simulink library "cmd_command_shaper_lib"  (R2016b)
settings: Solver=ode45  StartTime=0.0  StopTime=10.0  RelTol=1e-3  EnableMultiTasking=on
libraries: math_utils x4
settings Model: Creator=rhnakamu  LastModifiedBy=jfusco1
settings DataIOCC: LimitDataPoints=on  SaveFormat=Array
settings OptimizationCC: LifeSpan=inf
settings DebuggingCC: AllowSymbolicDim=off  SFUnexpectedBacktrackingDiag=warning  SFNoUnconditionalDefaultTransitionDiag=warning  SFExecutionAtInitializationDiag=none
settings HardwareCC: ProdBitPerPointer=32  ProdBitPerSizeT=32  ProdBitPerPtrDiffT=32  ProdLargestAtomicFloat=None  ProdIntDivRoundTo=Undefined  ProdEndianess=Unspecified  ProdWordSize=32  ProdHWDeviceType=32-bit Generic
settings ModelReferenceCC: PropagateSignalLabelsOutOfModel=off
settings GRTTargetCC: TargetLangStandard=C89/C90 (ANSI)  GeneratePreprocessorConditionals=Disable all
settings ConfigComp: CovMetricSettings=dw  CovHtmlReporting=on  CovSaveCumulativeToWorkspaceVar=on  CovSaveSingleToWorkspaceVar=on  CovExternalEMLEnable=off

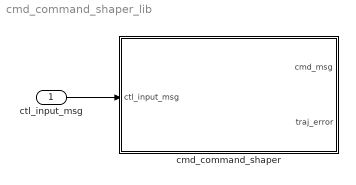
== system cmd_command_shaper_lib ==
  ctl_input_msg : Inport  OutDataTypeStr=Bus: ctl_input_msg
  cmd_command_shaper : Subsystem
  wires:
  ctl_input_msg/1 -> cmd_command_shaper/1(ctl_input_msg)

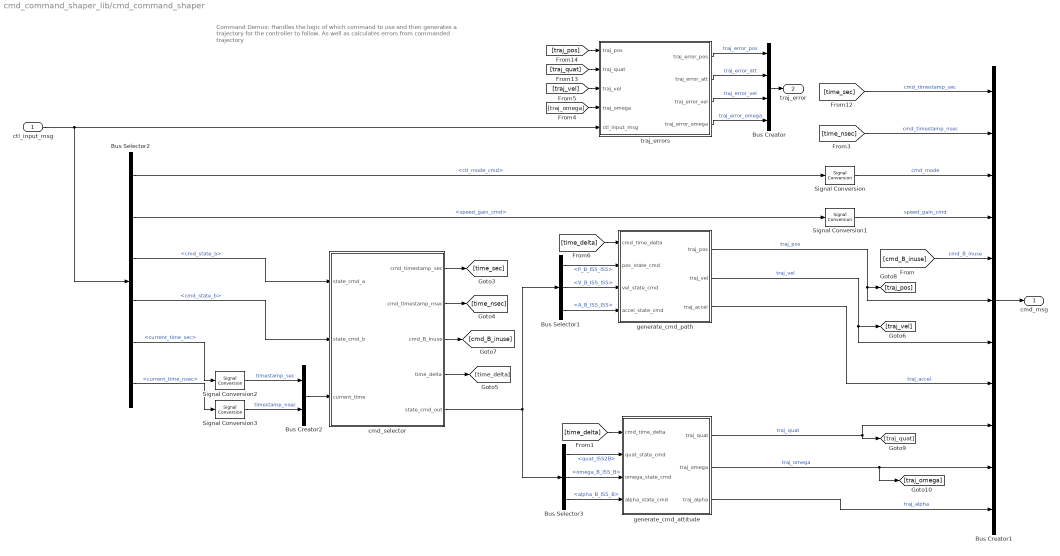
== system cmd_command_shaper_lib/cmd_command_shaper ==
  note: Command Demux:
      | Handles the logic of which command to use and then generates a trajectory for the controller to follow.
      | As well as calculates errors from commanded trajectory
  ctl_input_msg : Inport  OutDataTypeStr=Bus: ctl_input_msg
  Bus Creator : BusCreator  Inputs=4
  Bus Creator1 : BusCreator  Inputs=11  OutDataTypeStr=Bus: cmd_msg  NonVirtualBus=on
  Bus Creator2 : BusCreator  Inputs=2  OutDataTypeStr=Bus: ex_time_msg  NonVirtualBus=on
  Bus Selector1 : BusSelector  OutputSignals=P_B_ISS_ISS,V_B_ISS_ISS,A_B_ISS_ISS
  Bus Selector2 : BusSelector  OutputSignals=ctl_mode_cmd,speed_gain_cmd,cmd_state_a,cmd_state_b,current_time_sec,current_time_nsec
  Bus Selector3 : BusSelector  OutputSignals=quat_ISS2B,omega_B_ISS_B,alpha_B_ISS_B
  Signal Conversion{,1..3} (4 alike) : SignalConversion  OverrideOpt=off
  cmd_selector : Subsystem
  generate_cmd_attitude : Subsystem
  generate_cmd_path : Subsystem
  traj_errors : Subsystem
  cmd_msg : Outport  OutDataTypeStr=Bus: cmd_msg
  traj_error : Outport  Port=2
  wires:
  generate_cmd_attitude/1(traj_quat) -> Bus Creator1/9, [traj_quat]  "traj_quat"
  generate_cmd_attitude/2(traj_omega) -> [traj_omega], Bus Creator1/10  "traj_omega"
  generate_cmd_attitude/3(traj_alpha) -> Bus Creator1/11  "traj_alpha"
  generate_cmd_path/2(traj_vel) -> Bus Creator1/7, [traj_vel]  "traj_vel"
  generate_cmd_path/3(traj_accel) -> Bus Creator1/8  "traj_accel"
  generate_cmd_path/1(traj_pos) -> Bus Creator1/6, [traj_pos]  "traj_pos"
  [cmd_B_inuse] -> Bus Creator1/5  "cmd_B_inuse"
  cmd_selector/3(cmd_B_inuse) -> [cmd_B_inuse]
  [traj_pos] -> traj_errors/1(traj_pos)
  [traj_quat] -> traj_errors/2(traj_quat)
  Signal Conversion/1 -> Bus Creator1/3  "cmd_mode"
  Bus Selector2/1 -> Signal Conversion/1  "<ctl_mode_cmd>"
  [time_nsec] -> Bus Creator1/2  "cmd_timestamp_nsec"
  [time_sec] -> Bus Creator1/1  "cmd_timestamp_sec"
  Bus Creator1/1 -> cmd_msg/1
  Bus Creator2/1 -> cmd_selector/3(current_time)
  cmd_selector/4(time_delta) -> [time_delta]
  [time_delta] -> generate_cmd_path/1(cmd_time_delta)
  cmd_selector/1(cmd_timestamp_sec) -> [time_sec]
  cmd_selector/2(cmd_timestamp_nsec) -> [time_nsec]
  ctl_input_msg/1 -> traj_errors/5(ctl_input_msg), Bus Selector2/1
  cmd_selector/5(state_cmd_out) -> Bus Selector1/1, Bus Selector3/1
  [traj_vel] -> traj_errors/3(traj_vel)
  [traj_omega] -> traj_errors/4(traj_omega)
  traj_errors/1(traj_error_pos) -> Bus Creator/1  "traj_error_pos"
  traj_errors/2(traj_error_att) -> Bus Creator/2  "traj_error_att"
  traj_errors/3(traj_error_vel) -> Bus Creator/3  "traj_error_vel"
  traj_errors/4(traj_error_omega) -> Bus Creator/4  "traj_error_omega"
  Bus Creator/1 -> traj_error/1
  Bus Selector1/2 -> generate_cmd_path/3(vel_state_cmd)  "<V_B_ISS_ISS>"
  Bus Selector1/1 -> generate_cmd_path/2(pos_state_cmd)  "<P_B_ISS_ISS>"
  Bus Selector1/3 -> generate_cmd_path/4(accel_state_cmd)  "<A_B_ISS_ISS>"
  [time_delta] -> generate_cmd_attitude/1(cmd_time_delta)
  Bus Selector3/2 -> generate_cmd_attitude/3(omega_state_cmd)  "<omega_B_ISS_B>"
  Bus Selector3/1 -> generate_cmd_attitude/2(quat_state_cmd)  "<quat_ISS2B>"
  Bus Selector3/3 -> generate_cmd_attitude/4(alpha_state_cmd)  "<alpha_B_ISS_B>"
  Bus Selector2/3 -> cmd_selector/1(state_cmd_a)  "<cmd_state_a>"
  Bus Selector2/4 -> cmd_selector/2(state_cmd_b)  "<cmd_state_b>"
  Signal Conversion1/1 -> Bus Creator1/4  "speed_gain_cmd"
  Bus Selector2/2 -> Signal Conversion1/1  "<speed_gain_cmd>"
  Signal Conversion2/1 -> Bus Creator2/1  "timestamp_sec"
  Signal Conversion3/1 -> Bus Creator2/2  "timestamp_nsec"
  Bus Selector2/5 -> Signal Conversion2/1  "<current_time_sec>"
  Bus Selector2/6 -> Signal Conversion3/1  "<current_time_nsec>"

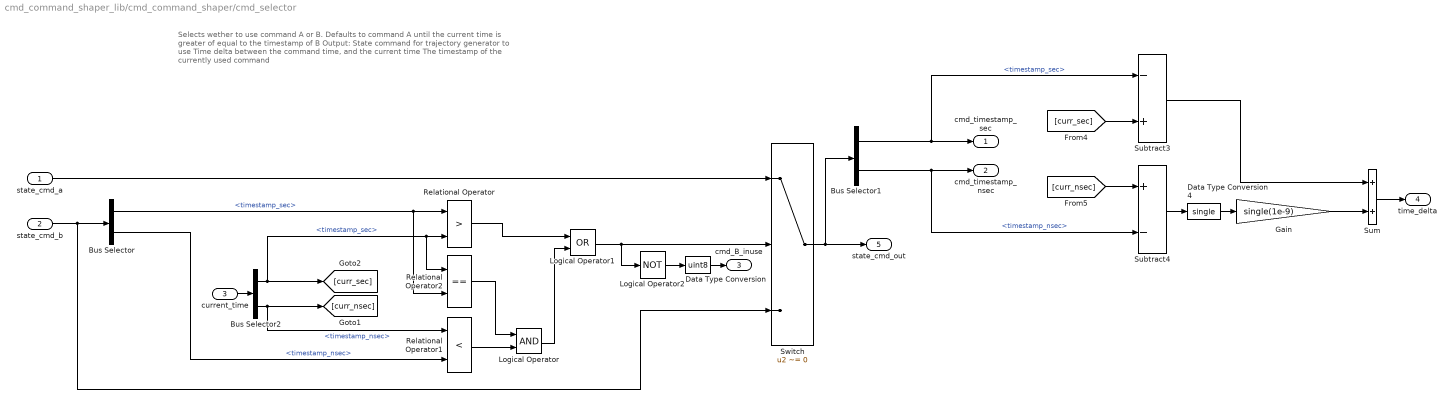
== system cmd_command_shaper_lib/cmd_command_shaper/cmd_selector ==
  note: Selects wether to use command A or B.
      | Defaults to command A until the current time is greater of equal to the timestamp of B
      |
      | Output:
      | 	State command for trajectory generator to use
      | 	Time delta between the command time, and the current time
      | 	The timestamp of the currently used command
  state_cmd_a : Inport
  state_cmd_b : Inport  Port=2
  current_time : Inport  Port=3
  Bus Selector : BusSelector  OutputSignals=timestamp_sec,timestamp_nsec
  Bus Selector1 : BusSelector  OutputSignals=timestamp_sec,timestamp_nsec
  Bus Selector2 : BusSelector  OutputSignals=timestamp_sec,timestamp_nsec
  Data Type Conversion : DataTypeConversion  OutDataTypeStr=uint8
  Data Type Conversion4 : DataTypeConversion  OutDataTypeStr=single
  Gain : Gain  Gain=single(1e-9)
  Logical Operator : Logic  AllPortsSameDT=off  OutDataTypeStr=boolean
  Logical Operator1 : Logic  Operator=OR  AllPortsSameDT=off  OutDataTypeStr=boolean
  Logical Operator2 : Logic  Operator=NOT  AllPortsSameDT=off  OutDataTypeStr=boolean
  Relational Operator : RelationalOperator  Operator=>  OutDataTypeStr=boolean  RndMeth=Nearest
  Relational Operator1 : RelationalOperator  Operator=<  OutDataTypeStr=boolean  RndMeth=Nearest
  Relational Operator2 : RelationalOperator  Operator===  OutDataTypeStr=boolean  RndMeth=Nearest
  Subtract3 : Sum  Inputs=-+  OutDataTypeStr=int32
      settings: AttributesFormatString=Out Type: %<OutDataTypeStr>
  Subtract4 : Sum  Inputs=+-  OutDataTypeStr=int32
      settings: AttributesFormatString=Out Type: %<OutDataTypeStr>
  Sum : Sum
  Switch : Switch  Criteria=u2 ~= 0
  cmd_timestamp_sec : Outport
  cmd_timestamp_nsec : Outport  Port=2
  cmd_B_inuse : Outport  Port=3
  time_delta : Outport  Port=4
  state_cmd_out : Outport  Port=5
  wires:
  Data Type Conversion/1 -> cmd_B_inuse/1
  Logical Operator2/1 -> Data Type Conversion/1
  Bus Selector1/2 -> cmd_timestamp_nsec/1, Subtract4/2  "<timestamp_nsec>"
  Bus Selector1/1 -> cmd_timestamp_sec/1, Subtract3/1  "<timestamp_sec>"
  Bus Selector/2 -> Relational Operator1/2  "<timestamp_nsec>"
  Bus Selector/1 -> Relational Operator/1, Relational Operator2/2  "<timestamp_sec>"
  Logical Operator1/1 -> Switch/2, Logical Operator2/1
  Subtract4/1 -> Data Type Conversion4/1
  [curr_sec] -> Subtract3/2
  [curr_nsec] -> Subtract4/1
  Sum/1 -> time_delta/1
  Data Type Conversion4/1 -> Gain/1
  Gain/1 -> Sum/2
  Subtract3/1 -> Sum/1
  Switch/1 -> Bus Selector1/1, state_cmd_out/1
  current_time/1 -> Bus Selector2/1
  Relational Operator/1 -> Logical Operator1/1
  Logical Operator/1 -> Logical Operator1/2
  Relational Operator2/1 -> Logical Operator/1
  Relational Operator1/1 -> Logical Operator/2
  Bus Selector2/1 -> [curr_sec], Relational Operator/2, Relational Operator2/1  "<timestamp_sec>"
  Bus Selector2/2 -> [curr_nsec], Relational Operator1/1  "<timestamp_nsec>"
  state_cmd_a/1 -> Switch/1
  state_cmd_b/1 -> Bus Selector/1, Switch/3

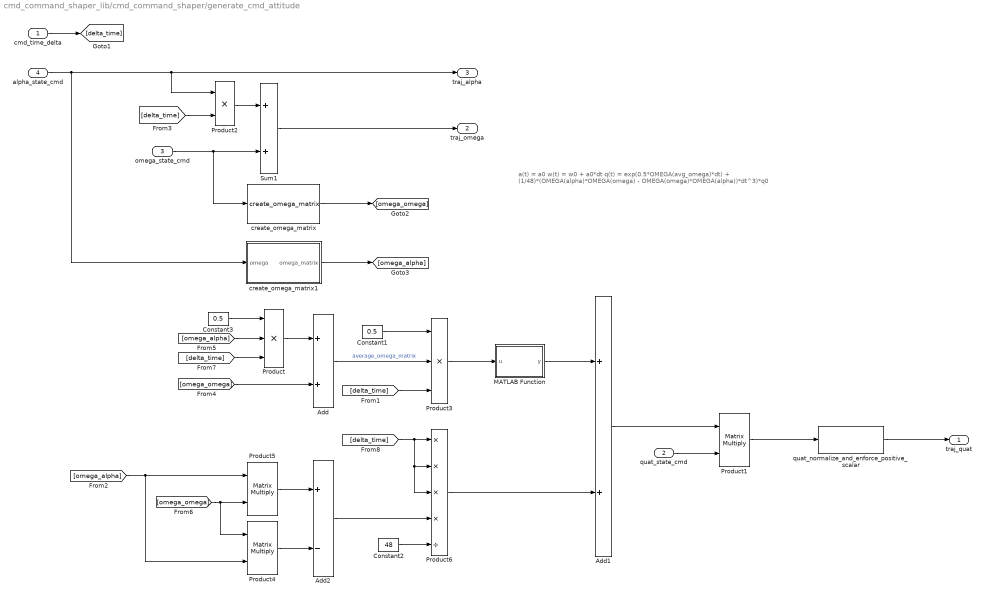
== system cmd_command_shaper_lib/cmd_command_shaper/generate_cmd_attitude ==
  note: a(t) = a0
      | w(t) = w0 + a0*dt
      | q(t) = exp(0.5*OMEGA(avg_omega)*dt) + (1/48)*(OMEGA(alpha)*OMEGA(omega) - OMEGA(omega)*OMEGA(alpha))*dt^3)*q0
  cmd_time_delta : Inport
  quat_state_cmd : Inport  Port=2
  omega_state_cmd : Inport  Port=3
  alpha_state_cmd : Inport  Port=4
  Add : Sum
  Add1 : Sum
  Add2 : Sum  Inputs=+-
  Constant1 : Constant  Value=0.5  OutDataTypeStr=Inherit: Inherit via back propagation
  Constant2 : Constant  Value=48  OutDataTypeStr=Inherit: Inherit via back propagation
  Constant3 : Constant  Value=0.5  OutDataTypeStr=Inherit: Inherit via back propagation
  MATLAB Function : MATLAB Function  TreatAsAtomicUnit=on
  Product : Product  Inputs=3
  Product1 : Product  Multiplication=Matrix(*)  RndMeth=Zero
  Product2 : Product  RndMeth=Zero  InputSameDT=on  OutDataTypeStr=Inherit: Same as first input
  Product3 : Product  Inputs=3
  Product4 : Product  Multiplication=Matrix(*)  RndMeth=Zero
  Product5 : Product  Multiplication=Matrix(*)  RndMeth=Zero
  Product6 : Product  Inputs=****/
  Sum1 : Sum
  create_omega_matrix : math_utils/create_omega_matrix  SystemSampleTime=-1
  create_omega_matrix1 : Subsystem
      mask Display: disp('\Omega(\omega)', 'tex', 'on');
  quat_normalize_and_enforce_positive_scalar : math_utils/quat_normalize_and_enforce_positive_scalar
  traj_quat : Outport
  traj_omega : Outport  Port=2
  traj_alpha : Outport  Port=3
  wires:
  Constant3/1 -> Product/1
  alpha_state_cmd/1 -> create_omega_matrix1/1(omega), Product2/1, traj_alpha/1
  Add1/1 -> Product1/1
  quat_state_cmd/1 -> Product1/2
  omega_state_cmd/1 -> create_omega_matrix/1, Sum1/2
  [delta_time] -> Product/3
  Product/1 -> Add/1
  Constant1/1 -> Product3/1
  Add/1 -> Product3/2  "average_omega_matrix"
  [delta_time] -> Product3/3
  Product3/1 -> MATLAB Function/1(u)
  MATLAB Function/1(y) -> Add1/1
  create_omega_matrix/1 -> [omega_omega]
  [omega_omega] -> Add/2
  [omega_alpha] -> Product/2
  create_omega_matrix1/1(omega_matrix) -> [omega_alpha]
  [omega_alpha] -> Product4/2, Product5/1
  Product5/1 -> Add2/1
  Product4/1 -> Add2/2
  [omega_omega] -> Product4/1, Product5/2
  Add2/1 -> Product6/4
  Constant2/1 -> Product6/5
  [delta_time] -> Product6/1, Product6/2, Product6/3
  Product6/1 -> Add1/2
  [delta_time] -> Product2/2
  cmd_time_delta/1 -> [delta_time]
  quat_normalize_and_enforce_positive_scalar/1 -> traj_quat/1
  Sum1/1 -> traj_omega/1
  Product2/1 -> Sum1/1
  Product1/1 -> quat_normalize_and_enforce_positive_scalar/1

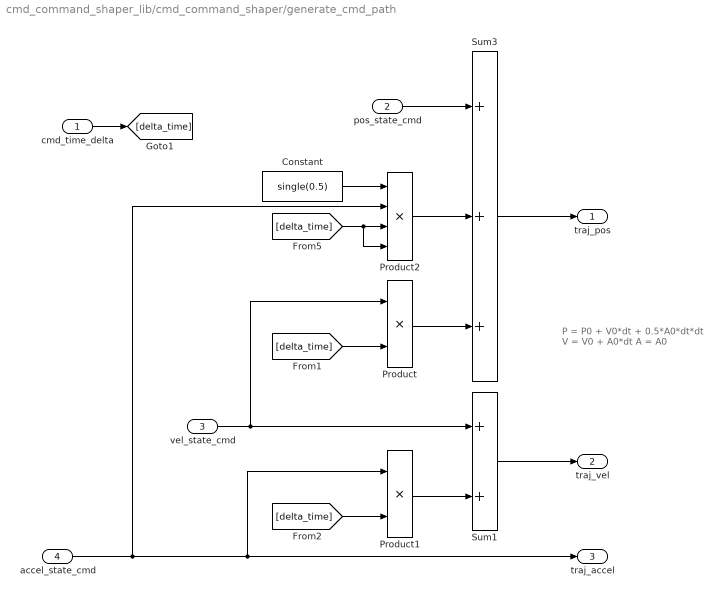
== system cmd_command_shaper_lib/cmd_command_shaper/generate_cmd_path ==
  note: P = P0 + V0*dt + 0.5*A0*dt*dt
      | V = V0 + A0*dt
      | A = A0
  cmd_time_delta : Inport
  pos_state_cmd : Inport  Port=2
  vel_state_cmd : Inport  Port=3
  accel_state_cmd : Inport  Port=4
  Constant : Constant  Value=single(0.5)
  Product : Product
  Product1 : Product
  Product2 : Product  Inputs=4
  Sum1 : Sum
  Sum3 : Sum  Inputs=+++
  traj_pos : Outport
  traj_vel : Outport  Port=2
  traj_accel : Outport  Port=3
  wires:
  [delta_time] -> Product/2
  [delta_time] -> Product1/2
  [delta_time] -> Product2/3, Product2/4
  cmd_time_delta/1 -> [delta_time]
  Constant/1 -> Product2/1
  Product2/1 -> Sum3/2
  Product/1 -> Sum3/3
  Product1/1 -> Sum1/2
  vel_state_cmd/1 -> Product/1, Sum1/1
  pos_state_cmd/1 -> Sum3/1
  accel_state_cmd/1 -> Product2/2, traj_accel/1, Product1/1
  Sum1/1 -> traj_vel/1
  Sum3/1 -> traj_pos/1

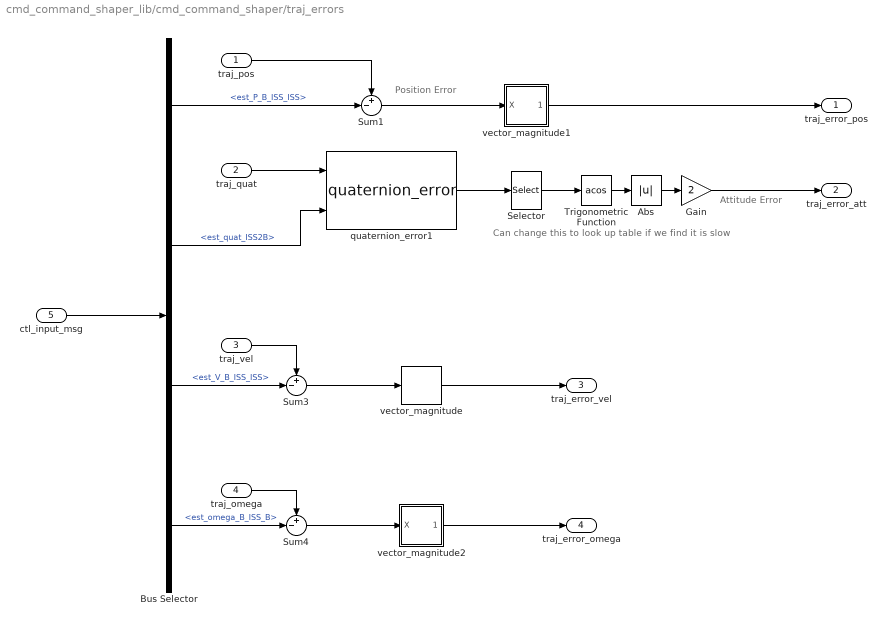
== system cmd_command_shaper_lib/cmd_command_shaper/traj_errors ==
  note: Can change this to look up table if we find it is slow
  note: Position Error
  note: Attitude Error
  traj_pos : Inport
  traj_quat : Inport  Port=2
  traj_vel : Inport  Port=3
  traj_omega : Inport  Port=4
  ctl_input_msg : Inport  Port=5  OutDataTypeStr=Bus: ctl_input_msg
  Abs : Abs
  Bus Selector : BusSelector  OutputSignals=est_P_B_ISS_ISS,est_quat_ISS2B,est_V_B_ISS_ISS,est_omega_B_ISS_B
  Gain : Gain  Gain=2
  Selector : Selector  InputPortWidth=4  IndexOptions=Index vector (dialog)  Indices=[4]  OutputSizes=1
  Sum1 : Sum  Inputs=+-|
  Sum3 : Sum  Inputs=+-|
  Sum4 : Sum  Inputs=+-|
  Trigonometric Function : Trigonometry  Operator=acos
  quaternion_error1 : math_utils/quaternion_error  SystemSampleTime=-1
  vector_magnitude : math_utils/vector_magnitude  SystemSampleTime=-1
  vector_magnitude1 : Subsystem
      mask Display: disp('|X|');
  vector_magnitude2 : Subsystem
      mask Display: disp('|X|');
  traj_error_pos : Outport
  traj_error_att : Outport  Port=2
  traj_error_vel : Outport  Port=3
  traj_error_omega : Outport  Port=4
  wires:
  ctl_input_msg/1 -> Bus Selector/1
  Bus Selector/1 -> Sum1/2  "<est_P_B_ISS_ISS>"
  Sum1/1 -> vector_magnitude1/1(X)
  traj_quat/1 -> quaternion_error1/1
  Bus Selector/2 -> quaternion_error1/2  "<est_quat_ISS2B>"
  quaternion_error1/1 -> Selector/1
  Trigonometric Function/1 -> Abs/1
  Selector/1 -> Trigonometric Function/1
  Abs/1 -> Gain/1
  traj_pos/1 -> Sum1/1
  vector_magnitude1/1(X_out) -> traj_error_pos/1
  Gain/1 -> traj_error_att/1
  traj_vel/1 -> Sum3/1
  Bus Selector/3 -> Sum3/2  "<est_V_B_ISS_ISS>"
  Sum3/1 -> vector_magnitude/1
  Sum4/1 -> vector_magnitude2/1(X)
  Bus Selector/4 -> Sum4/2  "<est_omega_B_ISS_B>"
  traj_omega/1 -> Sum4/1
  vector_magnitude/1 -> traj_error_vel/1
  vector_magnitude2/1(X_out) -> traj_error_omega/1

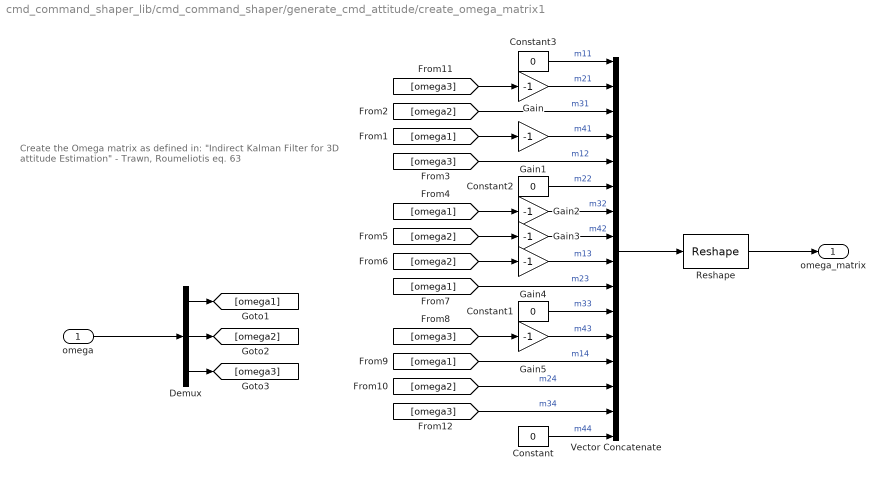
== system cmd_command_shaper_lib/cmd_command_shaper/generate_cmd_attitude/create_omega_matrix1 ==
  note: Create the Omega matrix as defined in:
      | "Indirect Kalman Filter for 3D attitude Estimation" - Trawn, Roumeliotis
      | eq. 63
  omega : Inport  PortDimensions=3
  Constant{,1..3} (4 alike) : Constant  Value=0  OutDataTypeStr=Inherit: Inherit via back propagation
  Demux : Demux  Outputs=3
  Gain{,1..5} (6 alike) : Gain  Gain=-1
  Reshape : Reshape  OutputDimensionality=Customize  OutputDimensions=[4,4]
  Vector Concatenate : Concatenate  NumInputs=16
  omega_matrix : Outport
  wires:
  omega/1 -> Demux/1
  Demux/1 -> [omega1]
  Demux/2 -> [omega2]
  Demux/3 -> [omega3]
  Vector Concatenate/1 -> Reshape/1
  Constant3/1 -> Vector Concatenate/1  "m11"
  Gain/1 -> Vector Concatenate/2  "m21"
  Constant2/1 -> Vector Concatenate/6  "m22"
  Gain1/1 -> Vector Concatenate/4  "m41"
  [omega2] -> Vector Concatenate/3  "m31"
  [omega3] -> Vector Concatenate/5  "m12"
  Gain2/1 -> Vector Concatenate/7  "m32"
  Gain3/1 -> Vector Concatenate/8  "m42"
  Gain4/1 -> Vector Concatenate/9  "m13"
  [omega1] -> Vector Concatenate/10  "m23"
  Constant1/1 -> Vector Concatenate/11  "m33"
  Constant/1 -> Vector Concatenate/16  "m44"
  Gain5/1 -> Vector Concatenate/12  "m43"
  [omega1] -> Vector Concatenate/13  "m14"
  [omega2] -> Vector Concatenate/14  "m24"
  [omega3] -> Vector Concatenate/15  "m34"
  Reshape/1 -> omega_matrix/1
  [omega3] -> Gain/1
  [omega1] -> Gain1/1
  [omega2] -> Gain3/1
  [omega1] -> Gain2/1
  [omega2] -> Gain4/1
  [omega3] -> Gain5/1

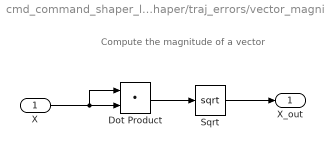
== system cmd_command_shaper_lib/cmd_command_shaper/traj_errors/vector_magnitude1 ==
  note: Compute the magnitude of a vector
  X : Inport
  Dot Product : DotProduct  InputSameDT=on  OutDataTypeStr=Inherit: Inherit via internal rule
  Sqrt : Sqrt  SaturateOnIntegerOverflow=on
  X_out : Outport
  wires:
  X/1 -> Dot Product/1, Dot Product/2
  Dot Product/1 -> Sqrt/1
  Sqrt/1 -> X_out/1

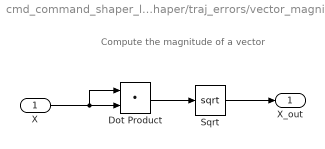
== system cmd_command_shaper_lib/cmd_command_shaper/traj_errors/vector_magnitude2 ==
  note: Compute the magnitude of a vector
  X : Inport
  Dot Product : DotProduct  InputSameDT=on  OutDataTypeStr=Inherit: Inherit via internal rule
  Sqrt : Sqrt  SaturateOnIntegerOverflow=on
  X_out : Outport
  wires:
  X/1 -> Dot Product/1, Dot Product/2
  Dot Product/1 -> Sqrt/1
  Sqrt/1 -> X_out/1

== matlab function cmd_command_shaper_lib/cmd_command_shaper/generate_cmd_attitude/MATLAB Function ==
  data: u input; y output
function y = expm(u)
%#codegen

y = expm(u);
